simulink model "Motor_Quadcopter_Combined_Current"  (R2016b)
settings: Solver=VariableStepAuto  StartTime=0.0  StopTime=500  RelTol=1e-3
libraries: simulink x36
(part 1 of 5)
settings Model: Creator=hermansoyfer  LastModifiedBy=cskulkar

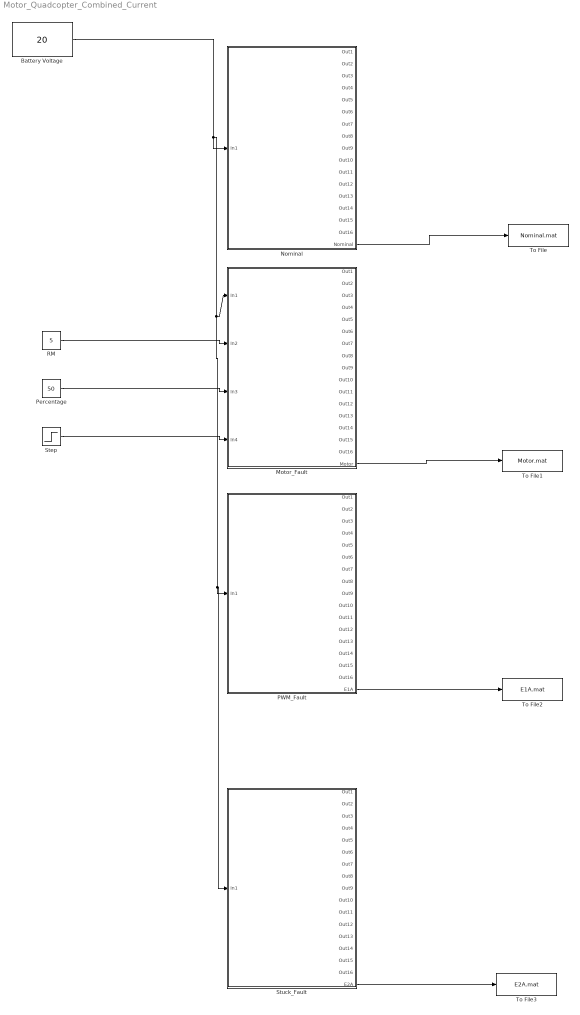
== system Motor_Quadcopter_Combined_Current ==
  Battery Voltage : Constant  Value=20
  Motor_Fault : Subsystem
  Nominal : Subsystem
  PWM_Fault : Subsystem
  Percentage : Constant  Value=50
  RM : Constant  Value=5
  Step : Step  Time=250  SampleTime=0
  Stuck_Fault : Subsystem
  To File : ToFile  Filename=Nominal.mat  MatrixName=Data
  To File1 : ToFile  Filename=Motor.mat  MatrixName=Data
  To File2 : ToFile  Filename=E1A.mat  MatrixName=Data
  To File3 : ToFile  Filename=E2A.mat  MatrixName=Data
  wires:
  Battery Voltage/1 -> Stuck_Fault/1(In1), PWM_Fault/1(In1), Motor_Fault/1(In1), Nominal/1(In1)
  Nominal/17(Nominal) -> To File/1
  Motor_Fault/17(Motor) -> To File1/1
  Percentage/1 -> Motor_Fault/3(In3)
  RM/1 -> Motor_Fault/2(In2)
  Step/1 -> Motor_Fault/4(In4)
  PWM_Fault/17(E1A) -> To File2/1
  Stuck_Fault/17(E2A) -> To File3/1

== system Motor_Quadcopter_Combined_Current/Motor_Fault ==
  In1 : Inport
  In2 : Inport  Port=2
  In3 : Inport  Port=3
  In4 : Inport  Port=4
  Add : Sum  Inputs=++++
  Add{1..4} (4 alike) : Sum
  Band-Limited White Noise1 : simulink/Sources/Band-Limited White Noise  Cov=[0.0001]  Ts=0.01  seed=[61]
  Band-Limited White Noise2 : simulink/Sources/Band-Limited White Noise  Cov=[0.0001]  Ts=0.01  seed=[678451]
  Band-Limited White Noise3 : simulink/Sources/Band-Limited White Noise  Cov=[0.0001]  Ts=0.01  seed=[95461]
  Band-Limited White Noise5 : simulink/Sources/Band-Limited White Noise  Cov=[0.0001]  Ts=0.01  seed=[34592]
  Gain : Gain  Gain=1/100
  Mux1 : Mux  Inputs=2
  Mux2 : Mux
  Mux3 : Mux
  Product : Product
  Product1 : Product
  Quadcopter_Arm1 : Subsystem
  Quadcopter_Arm3 : Subsystem
  Quadcopter_Arm4 : Subsystem
  Quatcopter_Arm2 : Subsystem
  Scope : Scope
  Scope1 : Scope  NumInputPorts=4
  Subsystem : Subsystem
  Subsystem1 : Subsystem
  Subsystem2 : Subsystem
  Subsystem3 : Subsystem
  Subsystem4 : Subsystem
  Subtract : Sum  Inputs=+-
  Out1 : Outport
  Out2 : Outport  Port=2
  Out3 : Outport  Port=3
  Out4 : Outport  Port=4
  Out5 : Outport  Port=5
  Out6 : Outport  Port=6
  Out7 : Outport  Port=7
  Out8 : Outport  Port=8
  Out9 : Outport  Port=9
  Out10 : Outport  Port=10
  Out11 : Outport  Port=11
  Out12 : Outport  Port=12
  Out13 : Outport  Port=13
  Out14 : Outport  Port=14
  Out15 : Outport  Port=15
  Out16 : Outport  Port=16
  Motor : Outport  Port=17
  wires:
  Quadcopter_Arm4/3(Out3) -> Out15/1
  Quatcopter_Arm2/4(Out4) -> Out8/1
  Quadcopter_Arm1/4(Out4) -> Out4/1
  In1/1 -> Quadcopter_Arm1/1(In1), Quatcopter_Arm2/1(In1), Quadcopter_Arm3/1(In1), Quadcopter_Arm4/1(In1)
  Quadcopter_Arm1/5(M1Current) -> Subsystem1/1(In1), Add/1
  Quatcopter_Arm2/5(M2Current) -> Subsystem2/1(In1), Add/2
  Quadcopter_Arm3/6(M3Current) -> Subsystem3/1(In1), Add/3
  Quadcopter_Arm4/6(M4Current) -> Subsystem4/1(In1), Add/4
  Quadcopter_Arm1/6(M1Voltage) -> Add1/1
  Quatcopter_Arm2/6(M2Voltatge) -> Add2/1
  Quadcopter_Arm3/5(M3Voltage) -> Add3/1
  Quadcopter_Arm4/5(M4Voltage) -> Add4/1
  Mux1/1 -> Motor/1
  Quadcopter_Arm4/4(Out4) -> Out16/1
  Quadcopter_Arm4/1(Out1) -> Out13/1
  Quadcopter_Arm4/2(Out2) -> Out14/1
  Quadcopter_Arm3/2(Out2) -> Out10/1
  Quatcopter_Arm2/2(Out2) -> Out6/1
  Quadcopter_Arm1/2(Out2) -> Out2/1
  Quadcopter_Arm3/3(Out3) -> Out11/1
  Quadcopter_Arm1/1(Out1) -> Out1/1
  Quatcopter_Arm2/3(Out3) -> Out7/1
  Quadcopter_Arm3/1(Out1) -> Out9/1
  Quatcopter_Arm2/1(Out1) -> Out5/1
  Quadcopter_Arm1/3(Out3) -> Out3/1
  Quadcopter_Arm3/4(Out4) -> Out12/1
  In4/1 -> Product1/2
  In2/1 -> Subtract/1, Product/1
  Product/1 -> Product1/1
  Product1/1 -> Subtract/2
  Subtract/1 -> Quadcopter_Arm1/2(Resistance)
  Gain/1 -> Product/2
  In3/1 -> Gain/1
  Band-Limited White Noise1/1 -> Add1/2
  Band-Limited White Noise2/1 -> Add2/2
  Band-Limited White Noise3/1 -> Add3/2
  Band-Limited White Noise5/1 -> Add4/2
  Add1/1 -> Scope1/1, Mux2/1
  Add2/1 -> Scope1/2, Mux2/2
  Add4/1 -> Scope1/4, Mux2/4
  Mux2/1 -> Mux1/1
  Subsystem/1(Out1) -> Scope/1
  Add/1 -> Subsystem/1(In1)
  Subsystem1/1(Out1) -> Mux3/1
  Subsystem2/1(Out1) -> Mux3/2
  Subsystem3/1(Out1) -> Mux3/3
  Subsystem4/1(Out1) -> Mux3/4
  Mux3/1 -> Mux1/2
  Add3/1 -> Scope1/3, Mux2/3

== system Motor_Quadcopter_Combined_Current/Nominal ==
  In1 : Inport
  Add : Sum  Inputs=++++
  Add{1..9} (9 alike) : Sum
  Band-Limited White Noise : simulink/Sources/Band-Limited White Noise  Cov=[0.0001]  Ts=0.01  seed=[23341]
  Band-Limited White Noise1 : simulink/Sources/Band-Limited White Noise  Cov=[0.0001]  Ts=0.01  seed=[322431]
  Band-Limited White Noise2 : simulink/Sources/Band-Limited White Noise  Cov=[0.0001]  Ts=0.01  seed=[685331]
  Band-Limited White Noise3 : simulink/Sources/Band-Limited White Noise  Cov=[0.0001]  Ts=0.01  seed=[456]
  Band-Limited White Noise4 : simulink/Sources/Band-Limited White Noise  Cov=[0.0001]  Ts=0.01  seed=[25561]
  Band-Limited White Noise5 : simulink/Sources/Band-Limited White Noise  Cov=[0.0001]  Ts=0.01  seed=[55321]
  Band-Limited White Noise6 : simulink/Sources/Band-Limited White Noise  Cov=[0.0005]  Ts=0.01  seed=[3452]
  Band-Limited White Noise7 : simulink/Sources/Band-Limited White Noise  Cov=[0.0002]  Ts=0.01  seed=[255]
  Band-Limited White Noise8 : simulink/Sources/Band-Limited White Noise  Cov=[0.0001]  Ts=0.01  seed=[61244]
  Mux : Mux
  Mux1 : Mux  Inputs=2
  Mux2 : Mux
  Quadcopter_Arm1 : Subsystem
  Quadcopter_Arm3 : Subsystem
  Quadcopter_Arm4 : Subsystem
  Quatcopter_Arm2 : Subsystem
  Scope : Scope
  Scope1 : Scope
  Scope2 : Scope
  Out1 : Outport
  Out2 : Outport  Port=2
  Out3 : Outport  Port=3
  Out4 : Outport  Port=4
  Out5 : Outport  Port=5
  Out6 : Outport  Port=6
  Out7 : Outport  Port=7
  Out8 : Outport  Port=8
  Out9 : Outport  Port=9
  Out10 : Outport  Port=10
  Out11 : Outport  Port=11
  Out12 : Outport  Port=12
  Out13 : Outport  Port=13
  Out14 : Outport  Port=14
  Out15 : Outport  Port=15
  Out16 : Outport  Port=16
  Nominal : Outport  Port=17
  wires:
  Quadcopter_Arm4/3(Out3) -> Out15/1
  Quatcopter_Arm2/4(Out4) -> Out8/1
  Quadcopter_Arm1/4(Out4) -> Out4/1
  In1/1 -> Quadcopter_Arm1/1(In1), Quatcopter_Arm2/1(In1), Quadcopter_Arm3/1(In1), Quadcopter_Arm4/1(In1)
  Quadcopter_Arm1/5(M1Current) -> Add6/1, Add/1
  Quatcopter_Arm2/5(M2Current) -> Add7/1, Add/2
  Quadcopter_Arm3/6(M3Current) -> Add9/1, Add8/1, Add/3
  Quadcopter_Arm4/6(M4Current) -> Add/4
  Quadcopter_Arm1/6(M1Voltage) -> Add1/1
  Quatcopter_Arm2/6(M2Voltatge) -> Add2/1
  Quadcopter_Arm3/5(M3Voltage) -> Add3/2
  Quadcopter_Arm4/5(M4Voltage) -> Add4/1
  Mux1/1 -> Nominal/1
  Quadcopter_Arm4/4(Out4) -> Out16/1
  Quadcopter_Arm4/1(Out1) -> Out13/1
  Quadcopter_Arm4/2(Out2) -> Out14/1
  Quadcopter_Arm3/2(Out2) -> Out10/1
  Quatcopter_Arm2/2(Out2) -> Out6/1
  Quadcopter_Arm1/2(Out2) -> Out2/1
  Quadcopter_Arm3/3(Out3) -> Out11/1
  Quadcopter_Arm1/1(Out1) -> Out1/1
  Quatcopter_Arm2/3(Out3) -> Out7/1
  Quadcopter_Arm3/1(Out1) -> Out9/1
  Quatcopter_Arm2/1(Out1) -> Out5/1
  Quadcopter_Arm1/3(Out3) -> Out3/1
  Quadcopter_Arm3/4(Out4) -> Out12/1
  Band-Limited White Noise/1 -> Add1/2
  Band-Limited White Noise1/1 -> Add2/2
  Band-Limited White Noise2/1 -> Add3/1
  Add1/1 -> Mux/1
  Add2/1 -> Mux/2
  Add3/1 -> Mux/3
  Add4/1 -> Mux/4
  Mux/1 -> Scope/1, Mux1/1
  Add/1 -> Add5/1
  Band-Limited White Noise4/1 -> Add5/2
  Add5/1 -> Scope1/1
  Band-Limited White Noise3/1 -> Add4/2
  Band-Limited White Noise5/1 -> Add6/2
  Add6/1 -> Mux2/1
  Band-Limited White Noise6/1 -> Add7/2
  Add7/1 -> Mux2/2
  Band-Limited White Noise7/1 -> Add8/2
  Add8/1 -> Mux2/3
  Add9/1 -> Mux2/4
  Band-Limited White Noise8/1 -> Add9/2
  Mux2/1 -> Scope2/1, Mux1/2

== system Motor_Quadcopter_Combined_Current/PWM_Fault ==
  In1 : Inport
  Add : Sum  Inputs=++++
  Add{1..4} (4 alike) : Sum
  Band-Limited White Noise{1..3,5} (4 alike) : simulink/Sources/Band-Limited White Noise  Cov=[0.0001]  Ts=0.01  seed=[46561]
  Mux1 : Mux  Inputs=2
  Mux2 : Mux
  Mux3 : Mux
  Quadcopter_Arm1 : Subsystem
  Quadcopter_Arm3 : Subsystem
  Quadcopter_Arm4 : Subsystem
  Quatcopter_Arm2 : Subsystem
  Scope : Scope
  Scope1 : Scope
  Subsystem : Subsystem
  Subsystem1 : Subsystem
  Subsystem2 : Subsystem
  Subsystem3 : Subsystem
  Subsystem4 : Subsystem
  Out1 : Outport
  Out2 : Outport  Port=2
  Out3 : Outport  Port=3
  Out4 : Outport  Port=4
  Out5 : Outport  Port=5
  Out6 : Outport  Port=6
  Out7 : Outport  Port=7
  Out8 : Outport  Port=8
  Out9 : Outport  Port=9
  Out10 : Outport  Port=10
  Out11 : Outport  Port=11
  Out12 : Outport  Port=12
  Out13 : Outport  Port=13
  Out14 : Outport  Port=14
  Out15 : Outport  Port=15
  Out16 : Outport  Port=16
  E1A : Outport  Port=17
  wires:
  Quadcopter_Arm4/3(Out3) -> Out15/1
  Quatcopter_Arm2/4(Out4) -> Out8/1
  Quadcopter_Arm1/4(Out4) -> Out4/1
  In1/1 -> Quadcopter_Arm1/1(In1), Quatcopter_Arm2/1(In1), Quadcopter_Arm3/1(In1), Quadcopter_Arm4/1(In1)
  Quadcopter_Arm1/5(M1Current) -> Subsystem1/1(In1), Add/1
  Quatcopter_Arm2/5(M2Current) -> Subsystem2/1(In1), Add/2
  Quadcopter_Arm3/6(M3Current) -> Subsystem3/1(In1), Add/3
  Quadcopter_Arm4/6(M4Current) -> Subsystem4/1(In1), Add/4
  Quadcopter_Arm1/6(M1Voltage) -> Add1/1
  Quatcopter_Arm2/6(M2Voltatge) -> Add2/1
  Quadcopter_Arm3/5(M3Voltage) -> Add3/1
  Quadcopter_Arm4/5(M4Voltage) -> Add4/1
  Mux1/1 -> E1A/1
  Quadcopter_Arm4/4(Out4) -> Out16/1
  Quadcopter_Arm4/1(Out1) -> Out13/1
  Quadcopter_Arm4/2(Out2) -> Out14/1
  Quadcopter_Arm3/2(Out2) -> Out10/1
  Quatcopter_Arm2/2(Out2) -> Out6/1
  Quadcopter_Arm1/2(Out2) -> Out2/1
  Quadcopter_Arm3/3(Out3) -> Out11/1
  Quadcopter_Arm1/1(Out1) -> Out1/1
  Quatcopter_Arm2/3(Out3) -> Out7/1
  Quadcopter_Arm3/1(Out1) -> Out9/1
  Quatcopter_Arm2/1(Out1) -> Out5/1
  Quadcopter_Arm1/3(Out3) -> Out3/1
  Quadcopter_Arm3/4(Out4) -> Out12/1
  Band-Limited White Noise1/1 -> Add1/2
  Band-Limited White Noise2/1 -> Add2/2
  Band-Limited White Noise3/1 -> Add3/2
  Band-Limited White Noise5/1 -> Add4/2
  Add1/1 -> Mux2/1
  Add2/1 -> Mux2/2
  Add3/1 -> Mux2/3
  Mux2/1 -> Scope/1, Mux1/1
  Add4/1 -> Mux2/4
  Subsystem/1(Out1) -> Scope1/1
  Add/1 -> Subsystem/1(In1)
  Subsystem1/1(Out1) -> Mux3/1
  Subsystem2/1(Out1) -> Mux3/2
  Subsystem3/1(Out1) -> Mux3/3
  Subsystem4/1(Out1) -> Mux3/4
  Mux3/1 -> Mux1/2

== system Motor_Quadcopter_Combined_Current/Stuck_Fault ==
  In1 : Inport
  Add : Sum  Inputs=++++
  Add{1..4} (4 alike) : Sum
  Band-Limited White Noise1 : simulink/Sources/Band-Limited White Noise  Cov=[0.0001]  Ts=0.01  seed=[678]
  Band-Limited White Noise2 : simulink/Sources/Band-Limited White Noise  Cov=[0.0001]  Ts=0.01  seed=[1111]
  Band-Limited White Noise3 : simulink/Sources/Band-Limited White Noise  Cov=[0.0001]  Ts=0.01  seed=[61]
  Band-Limited White Noise5 : simulink/Sources/Band-Limited White Noise  Cov=[0.0001]  Ts=0.01  seed=[4]
  Mux1 : Mux  Inputs=2
  Mux2 : Mux
  Mux3 : Mux
  Quadcopter_Arm1 : Subsystem
  Quadcopter_Arm3 : Subsystem
  Quadcopter_Arm4 : Subsystem
  Quatcopter_Arm2 : Subsystem
  Scope : Scope
  Scope1 : Scope
  Scope2 : Scope  NumInputPorts=4
  Subsystem : Subsystem
  Subsystem1 : Subsystem
  Subsystem2 : Subsystem
  Subsystem3 : Subsystem
  Subsystem4 : Subsystem
  Out1 : Outport
  Out2 : Outport  Port=2
  Out3 : Outport  Port=3
  Out4 : Outport  Port=4
  Out5 : Outport  Port=5
  Out6 : Outport  Port=6
  Out7 : Outport  Port=7
  Out8 : Outport  Port=8
  Out9 : Outport  Port=9
  Out10 : Outport  Port=10
  Out11 : Outport  Port=11
  Out12 : Outport  Port=12
  Out13 : Outport  Port=13
  Out14 : Outport  Port=14
  Out15 : Outport  Port=15
  Out16 : Outport  Port=16
  E2A : Outport  Port=17
  wires:
  Quadcopter_Arm4/3(Out3) -> Out15/1
  Quatcopter_Arm2/4(Out4) -> Out8/1
  Quadcopter_Arm1/4(Out4) -> Out4/1
  In1/1 -> Quadcopter_Arm1/1(In1), Quatcopter_Arm2/1(In1), Quadcopter_Arm3/1(In1), Quadcopter_Arm4/1(In1)
  Quadcopter_Arm1/5(M1Current) -> Subsystem1/1(In1), Add/1
  Quatcopter_Arm2/5(M2Current) -> Subsystem2/1(In1), Add/2
  Quadcopter_Arm3/6(M3Current) -> Subsystem3/1(In1), Add/3
  Quadcopter_Arm4/6(M4Current) -> Subsystem4/1(In1), Add/4
  Quadcopter_Arm1/6(M1Voltage) -> Add1/1
  Quadcopter_Arm4/4(Out4) -> Out16/1
  Quadcopter_Arm4/1(Out1) -> Out13/1
  Quadcopter_Arm4/2(Out2) -> Out14/1
  Quadcopter_Arm3/2(Out2) -> Out10/1
  Quatcopter_Arm2/2(Out2) -> Out6/1
  Quadcopter_Arm1/2(Out2) -> Out2/1
  Quadcopter_Arm3/3(Out3) -> Out11/1
  Quadcopter_Arm1/1(Out1) -> Out1/1
  Quatcopter_Arm2/3(Out3) -> Out7/1
  Quadcopter_Arm3/1(Out1) -> Out9/1
  Quatcopter_Arm2/1(Out1) -> Out5/1
  Quadcopter_Arm1/3(Out3) -> Out3/1
  Quadcopter_Arm3/4(Out4) -> Out12/1
  Band-Limited White Noise1/1 -> Add1/2
  Band-Limited White Noise2/1 -> Add2/2
  Band-Limited White Noise3/1 -> Add3/2
  Band-Limited White Noise5/1 -> Add4/2
  Quatcopter_Arm2/6(M2Voltatge) -> Add2/1
  Quadcopter_Arm3/5(M3Voltage) -> Add3/1
  Quadcopter_Arm4/5(M4Voltage) -> Add4/1
  Add1/1 -> Mux2/1
  Add2/1 -> Mux2/2
  Add3/1 -> Mux2/3
  Add4/1 -> Mux2/4
  Mux2/1 -> Mux1/1
  Mux1/1 -> Scope/1, E2A/1
  Subsystem/1(Out1) -> Scope1/1
  Add/1 -> Subsystem/1(In1)
  Subsystem1/1(Out1) -> Scope2/2, Mux3/1
  Subsystem2/1(Out1) -> Scope2/1, Mux3/2
  Subsystem3/1(Out1) -> Scope2/3, Mux3/3
  Subsystem4/1(Out1) -> Scope2/4, Mux3/4
  Mux3/1 -> Mux1/2

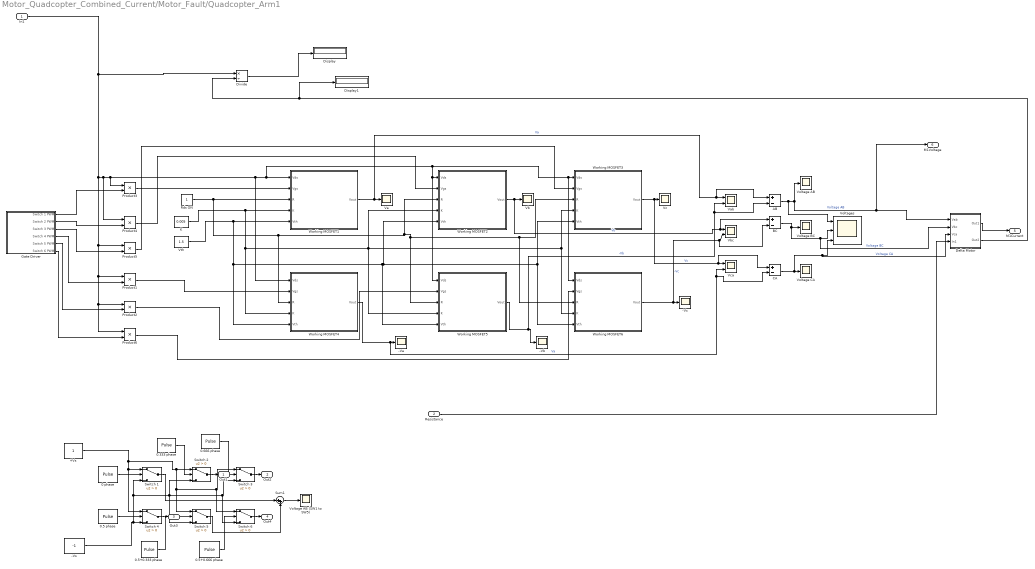
== system Motor_Quadcopter_Combined_Current/Motor_Fault/Quadcopter_Arm1 ==
  In1 : Inport
  Resistance : Inport  Port=2
  +Vs : Constant
  -Va : Scope
  -Vb : Scope
  -Vc : Scope
  -Vs : Constant  Value=-1
  0 phase : DiscretePulseGenerator  PulseType=Time based  Period=1  PulseWidth=50
  0.333 phase : DiscretePulseGenerator  PulseType=Time based  Period=1  PulseWidth=50  PhaseDelay=1/3
  0.5 phase : DiscretePulseGenerator  PulseType=Time based  Period=1  PulseWidth=50  PhaseDelay=.5
  0.5+0.333 phase : DiscretePulseGenerator  PulseType=Time based  Period=1  PulseWidth=50  PhaseDelay=0.5 + 1/3
  0.5+0.666 phase : DiscretePulseGenerator  PulseType=Time based  Period=1  PulseWidth=50  PhaseDelay=2/3+0.5
  0.666 phase : DiscretePulseGenerator  PulseType=Time based  Period=1  PulseWidth=50  PhaseDelay=2/3
  AB : Sum  Inputs=+-
  BC : Sum  Inputs=+-
  CA : Sum  Inputs=+-
  Delta Motor : Subsystem
  Display : Display
  Display1 : Display
  Divide : Product  Inputs=*/
  Gate Driver : Subsystem
  K : Constant  Value=0.005
  Product{1..6} (6 alike) : Product
  Rds ON : Constant
  Sum1 : Sum  Inputs=|++
  Switch {1..6} (6 alike) : Switch  Criteria=u2 > Threshold
  Va : Scope
  Vab : Scope  NumInputPorts=2
  Vb : Scope
  Vbc : Scope  NumInputPorts=2
  Vc : Scope
  Vca : Scope  NumInputPorts=2
  Voltage AB : Scope
  Voltage AB (SW1 to SW5) : Scope
  Voltage BC : Scope
  Voltage CA : Scope
  Voltages : Scope  NumInputPorts=3
  Vth : Constant  Value=1.5
  Working MOSFET1 : MATLAB Function  TreatAsAtomicUnit=on
  Working MOSFET2 : MATLAB Function  TreatAsAtomicUnit=on
  Working MOSFET3 : MATLAB Function  TreatAsAtomicUnit=on
  Working MOSFET4 : MATLAB Function  TreatAsAtomicUnit=on
  Working MOSFET5 : MATLAB Function  TreatAsAtomicUnit=on
  Working MOSFET6 : MATLAB Function  TreatAsAtomicUnit=on
  Out1 : Outport
  Out2 : Outport  Port=2
  Out3 : Outport  Port=3
  Out4 : Outport  Port=4
  M1Current : Outport  Port=5
  M1Voltage : Outport  Port=6
  wires:
  Switch 5/1 -> Sum1/2
  Working MOSFET4/1(Vout) -> CA/2, Vca/2, -Va/1  "Va"
  Working MOSFET6/1(Vout) -> BC/2, Vbc/2, -Vc/1  "-Vc"
  AB/1 -> Voltages/1, M1Voltage/1, Delta Motor/1(Vab), Voltage AB/1  "Voltage AB"
  In1/1 -> Divide/1, Product6/1, Product2/1, Product1/1, Product5/1, Product4/1, Working MOSFET4/1(Vds), Working MOSFET6/1(Vds), Working MOSFET3/1(Vds), Working MOSFET5/1(Vds), Working MOSFET2/1(Vds), Working MOSFET1/1(Vds), Product3/1
  K/1 -> Working MOSFET4/4(K), Working MOSFET5/4(K), Working MOSFET2/4(K), Working MOSFET6/4(K), Working MOSFET3/4(K), Working MOSFET1/4(K)
  Product5/1 -> Working MOSFET3/2(Vgs)
  0.5+0.333 phase/1 -> Switch 5/2
  Gate Driver/3(Switch 3 PWM) -> Product5/2
  Gate Driver/6(Switch 6 PWM) -> Product6/2
  Working MOSFET5/1(Vout) -> AB/2, Vab/2, -Vb/1  "-Vb"
  Gate Driver/5(Switch 5 PWM) -> Product2/2
  Working MOSFET1/1(Vout) -> AB/1, Vab/1, Va/1  "Va"
  0 phase/1 -> Switch 1/2
  Gate Driver/2(Switch 2 PWM) -> Product4/2
  Gate Driver/4(Switch 4 PWM) -> Product1/2
  BC/1 -> Delta Motor/2(Vbc), Voltages/2, Voltage BC/1  "Voltage BC"
  CA/1 -> Delta Motor/3(Vca), Voltages/3, Voltage CA/1  "Voltage CA"
  Working MOSFET3/1(Vout) -> CA/1, Vca/1, Vc/1  "Vc"
  Gate Driver/1(Switch 1 PWM) -> Product3/2
  Vth/1 -> Working MOSFET4/5(Vth), Working MOSFET5/5(Vth), Working MOSFET2/5(Vth), Working MOSFET6/5(Vth), Working MOSFET3/5(Vth), Working MOSFET1/5(Vth)
  Product1/1 -> Working MOSFET4/2(Vgs)
  0.333 phase/1 -> Switch 2/2
  Sum1/1 -> Voltage AB (SW1 to SW5)/1
  0.5 phase/1 -> Switch 4/2
  Switch 1/1 -> Sum1/1
  Working MOSFET2/1(Vout) -> BC/1, Vbc/1, Vb/1  "Vb"
  Switch 6/1 -> Out4/1
  Switch 2/1 -> Out1/1
  Switch 4/1 -> Out3/1
  Product2/1 -> Working MOSFET5/2(Vgs)
  Switch 3/1 -> Out2/1
  +Vs/1 -> Switch 6/1, Switch 3/1, Switch 5/1, Switch 2/1, Switch 4/1, Switch 1/1
  0.666 phase/1 -> Switch 3/2
  0.5+0.666 phase/1 -> Switch 6/2
  -Vs/1 -> Switch 1/3, Switch 6/3, Switch 3/3, Switch 2/3, Switch 5/3, Switch 4/3
  Rds ON/1 -> Working MOSFET1/3(R), Working MOSFET4/3(R), Working MOSFET3/3(R), Working MOSFET6/3(R), Working MOSFET5/3(R), Working MOSFET2/3(R)
  Product4/1 -> Working MOSFET2/2(Vgs)
  Product3/1 -> Working MOSFET1/2(Vgs)
  Product6/1 -> Working MOSFET6/2(Vgs)
  Delta Motor/1(Out1) -> M1Current/1
  Divide/1 -> Display/1
  Delta Motor/2(Out2) -> Display1/1, Divide/2
  Resistance/1 -> Delta Motor/4(In1)

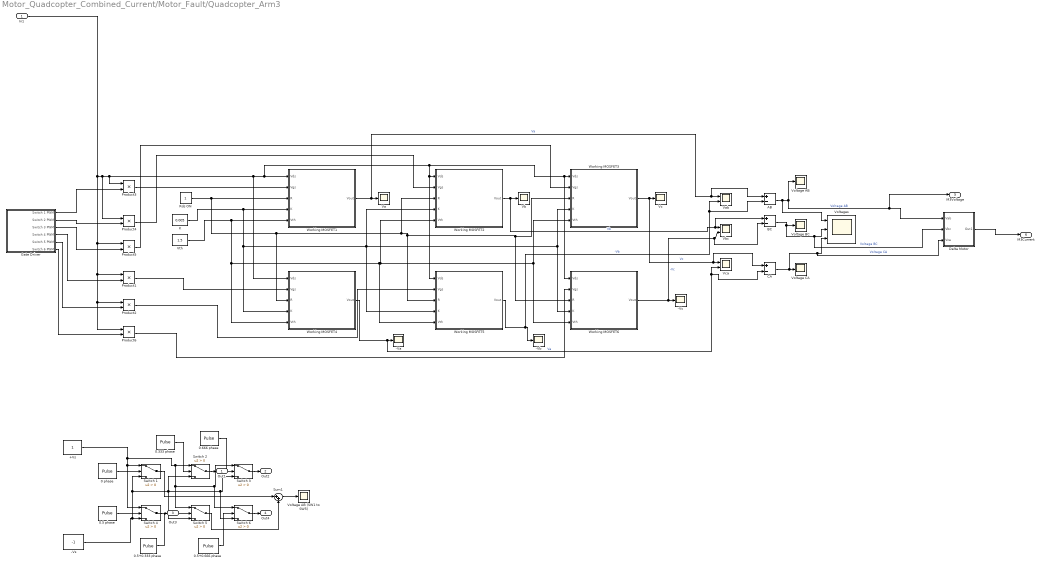
== system Motor_Quadcopter_Combined_Current/Motor_Fault/Quadcopter_Arm3 ==
  In1 : Inport
  +Vs : Constant
  -Va : Scope
  -Vb : Scope
  -Vc : Scope
  -Vs : Constant  Value=-1
  0 phase : DiscretePulseGenerator  PulseType=Time based  Period=1  PulseWidth=50
  0.333 phase : DiscretePulseGenerator  PulseType=Time based  Period=1  PulseWidth=50  PhaseDelay=1/3
  0.5 phase : DiscretePulseGenerator  PulseType=Time based  Period=1  PulseWidth=50  PhaseDelay=.5
  0.5+0.333 phase : DiscretePulseGenerator  PulseType=Time based  Period=1  PulseWidth=50  PhaseDelay=0.5 + 1/3
  0.5+0.666 phase : DiscretePulseGenerator  PulseType=Time based  Period=1  PulseWidth=50  PhaseDelay=2/3+0.5
  0.666 phase : DiscretePulseGenerator  PulseType=Time based  Period=1  PulseWidth=50  PhaseDelay=2/3
  AB : Sum  Inputs=+-
  BC : Sum  Inputs=+-
  CA : Sum  Inputs=+-
  Delta Motor : Subsystem
  Gate Driver : Subsystem
  K : Constant  Value=0.005
  Product{1..6} (6 alike) : Product
  Rds ON : Constant
  Sum1 : Sum  Inputs=|++
  Switch {1..6} (6 alike) : Switch  Criteria=u2 > Threshold
  Va : Scope
  Vab : Scope  NumInputPorts=2
  Vb : Scope
  Vbc : Scope  NumInputPorts=2
  Vc : Scope
  Vca : Scope  NumInputPorts=2
  Voltage AB : Scope
  Voltage AB (SW1 to SW5) : Scope
  Voltage BC : Scope
  Voltage CA : Scope
  Voltages : Scope  NumInputPorts=3
  Vth : Constant  Value=1.5
  Working MOSFET1 : MATLAB Function  TreatAsAtomicUnit=on
  Working MOSFET2 : MATLAB Function  TreatAsAtomicUnit=on
  Working MOSFET3 : MATLAB Function  TreatAsAtomicUnit=on
  Working MOSFET4 : MATLAB Function  TreatAsAtomicUnit=on
  Working MOSFET5 : MATLAB Function  TreatAsAtomicUnit=on
  Working MOSFET6 : MATLAB Function  TreatAsAtomicUnit=on
  Out1 : Outport
  Out2 : Outport  Port=2
  Out3 : Outport  Port=3
  Out4 : Outport  Port=4
  M3Voltage : Outport  Port=5
  M3Current : Outport  Port=6
  wires:
  Switch 5/1 -> Sum1/2
  Working MOSFET4/1(Vout) -> CA/2, Vca/2, -Va/1  "Va"
  Working MOSFET6/1(Vout) -> BC/2, Vbc/2, -Vc/1  "-Vc"
  AB/1 -> Voltages/1, M3Voltage/1, Delta Motor/1(Vab), Voltage AB/1  "Voltage AB"
  In1/1 -> Product6/1, Product2/1, Product1/1, Product5/1, Product4/1, Working MOSFET4/1(Vds), Working MOSFET6/1(Vds), Working MOSFET3/1(Vds), Working MOSFET5/1(Vds), Working MOSFET2/1(Vds), Working MOSFET1/1(Vds), Product3/1
  K/1 -> Working MOSFET4/4(K), Working MOSFET5/4(K), Working MOSFET2/4(K), Working MOSFET6/4(K), Working MOSFET3/4(K), Working MOSFET1/4(K)
  Product5/1 -> Working MOSFET3/2(Vgs)
  0.5+0.333 phase/1 -> Switch 5/2
  Gate Driver/3(Switch 3 PWM) -> Product5/2
  Gate Driver/6(Switch 6 PWM) -> Product6/2
  Working MOSFET5/1(Vout) -> AB/2, Vab/2, -Vb/1  "-Vb"
  Gate Driver/5(Switch 5 PWM) -> Product2/2
  Working MOSFET1/1(Vout) -> AB/1, Vab/1, Va/1  "Va"
  0 phase/1 -> Switch 1/2
  Gate Driver/2(Switch 2 PWM) -> Product4/2
  Gate Driver/4(Switch 4 PWM) -> Product1/2
  BC/1 -> Delta Motor/2(Vbc), Voltages/2, Voltage BC/1  "Voltage BC"
  CA/1 -> Delta Motor/3(Vca), Voltages/3, Voltage CA/1  "Voltage CA"
  Working MOSFET3/1(Vout) -> CA/1, Vca/1, Vc/1  "Vc"
  Gate Driver/1(Switch 1 PWM) -> Product3/2
  Vth/1 -> Working MOSFET4/5(Vth), Working MOSFET5/5(Vth), Working MOSFET2/5(Vth), Working MOSFET6/5(Vth), Working MOSFET3/5(Vth), Working MOSFET1/5(Vth)
  Product1/1 -> Working MOSFET4/2(Vgs)
  0.333 phase/1 -> Switch 2/2
  Sum1/1 -> Voltage AB (SW1 to SW5)/1
  0.5 phase/1 -> Switch 4/2
  Switch 1/1 -> Sum1/1
  Working MOSFET2/1(Vout) -> BC/1, Vbc/1, Vb/1  "Vb"
  Switch 6/1 -> Out4/1
  Switch 2/1 -> Out1/1
  Switch 4/1 -> Out3/1
  Product2/1 -> Working MOSFET5/2(Vgs)
  Switch 3/1 -> Out2/1
  +Vs/1 -> Switch 6/1, Switch 3/1, Switch 5/1, Switch 2/1, Switch 4/1, Switch 1/1
  0.666 phase/1 -> Switch 3/2
  0.5+0.666 phase/1 -> Switch 6/2
  -Vs/1 -> Switch 1/3, Switch 6/3, Switch 3/3, Switch 2/3, Switch 5/3, Switch 4/3
  Rds ON/1 -> Working MOSFET1/3(R), Working MOSFET4/3(R), Working MOSFET3/3(R), Working MOSFET6/3(R), Working MOSFET5/3(R), Working MOSFET2/3(R)
  Product4/1 -> Working MOSFET2/2(Vgs)
  Product3/1 -> Working MOSFET1/2(Vgs)
  Product6/1 -> Working MOSFET6/2(Vgs)
  Delta Motor/1(Out1) -> M3Current/1

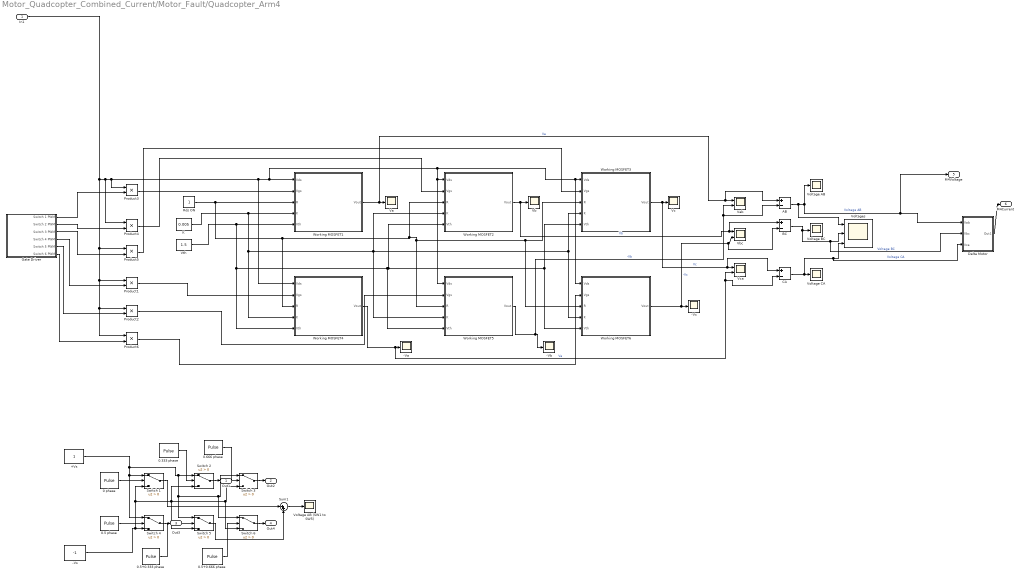
== system Motor_Quadcopter_Combined_Current/Motor_Fault/Quadcopter_Arm4 ==
  In1 : Inport
  +Vs : Constant
  -Va : Scope
  -Vb : Scope
  -Vc : Scope
  -Vs : Constant  Value=-1
  0 phase : DiscretePulseGenerator  PulseType=Time based  Period=1  PulseWidth=50
  0.333 phase : DiscretePulseGenerator  PulseType=Time based  Period=1  PulseWidth=50  PhaseDelay=1/3
  0.5 phase : DiscretePulseGenerator  PulseType=Time based  Period=1  PulseWidth=50  PhaseDelay=.5
  0.5+0.333 phase : DiscretePulseGenerator  PulseType=Time based  Period=1  PulseWidth=50  PhaseDelay=0.5 + 1/3
  0.5+0.666 phase : DiscretePulseGenerator  PulseType=Time based  Period=1  PulseWidth=50  PhaseDelay=2/3+0.5
  0.666 phase : DiscretePulseGenerator  PulseType=Time based  Period=1  PulseWidth=50  PhaseDelay=2/3
  AB : Sum  Inputs=+-
  BC : Sum  Inputs=+-
  CA : Sum  Inputs=+-
  Delta Motor : Subsystem
  Gate Driver : Subsystem
  K : Constant  Value=0.005
  Product{1..6} (6 alike) : Product
  Rds ON : Constant
  Sum1 : Sum  Inputs=|++
  Switch {1..6} (6 alike) : Switch  Criteria=u2 > Threshold
  Va : Scope
  Vab : Scope  NumInputPorts=2
  Vb : Scope
  Vbc : Scope  NumInputPorts=2
  Vc : Scope
  Vca : Scope  NumInputPorts=2
  Voltage AB : Scope
  Voltage AB (SW1 to SW5) : Scope
  Voltage BC : Scope
  Voltage CA : Scope
  Voltages : Scope  NumInputPorts=3
  Vth : Constant  Value=1.5
  Working MOSFET1 : MATLAB Function  TreatAsAtomicUnit=on
  Working MOSFET2 : MATLAB Function  TreatAsAtomicUnit=on
  Working MOSFET3 : MATLAB Function  TreatAsAtomicUnit=on
  Working MOSFET4 : MATLAB Function  TreatAsAtomicUnit=on
  Working MOSFET5 : MATLAB Function  TreatAsAtomicUnit=on
  Working MOSFET6 : MATLAB Function  TreatAsAtomicUnit=on
  Out1 : Outport
  Out2 : Outport  Port=2
  Out3 : Outport  Port=3
  Out4 : Outport  Port=4
  M4Voltage : Outport  Port=5
  M4Current : Outport  Port=6
  wires:
  Switch 5/1 -> Sum1/2
  Working MOSFET4/1(Vout) -> CA/2, Vca/2, -Va/1  "Va"
  Working MOSFET6/1(Vout) -> BC/2, Vbc/2, -Vc/1  "-Vc"
  AB/1 -> Voltages/1, M4Voltage/1, Delta Motor/1(Vab), Voltage AB/1  "Voltage AB"
  In1/1 -> Product6/1, Product2/1, Product1/1, Product5/1, Product4/1, Working MOSFET4/1(Vds), Working MOSFET6/1(Vds), Working MOSFET3/1(Vds), Working MOSFET5/1(Vds), Working MOSFET2/1(Vds), Working MOSFET1/1(Vds), Product3/1
  K/1 -> Working MOSFET4/4(K), Working MOSFET5/4(K), Working MOSFET2/4(K), Working MOSFET6/4(K), Working MOSFET3/4(K), Working MOSFET1/4(K)
  Product5/1 -> Working MOSFET3/2(Vgs)
  0.5+0.333 phase/1 -> Switch 5/2
  Gate Driver/3(Switch 3 PWM) -> Product5/2
  Gate Driver/6(Switch 6 PWM) -> Product6/2
  Working MOSFET5/1(Vout) -> AB/2, Vab/2, -Vb/1  "-Vb"
  Gate Driver/5(Switch 5 PWM) -> Product2/2
  Working MOSFET1/1(Vout) -> AB/1, Vab/1, Va/1  "Va"
  0 phase/1 -> Switch 1/2
  Gate Driver/2(Switch 2 PWM) -> Product4/2
  Gate Driver/4(Switch 4 PWM) -> Product1/2
  BC/1 -> Delta Motor/2(Vbc), Voltages/2, Voltage BC/1  "Voltage BC"
  CA/1 -> Delta Motor/3(Vca), Voltages/3, Voltage CA/1  "Voltage CA"
  Working MOSFET3/1(Vout) -> CA/1, Vca/1, Vc/1  "Vc"
  Gate Driver/1(Switch 1 PWM) -> Product3/2
  Vth/1 -> Working MOSFET4/5(Vth), Working MOSFET5/5(Vth), Working MOSFET2/5(Vth), Working MOSFET6/5(Vth), Working MOSFET3/5(Vth), Working MOSFET1/5(Vth)
  Product1/1 -> Working MOSFET4/2(Vgs)
  0.333 phase/1 -> Switch 2/2
  Sum1/1 -> Voltage AB (SW1 to SW5)/1
  0.5 phase/1 -> Switch 4/2
  Switch 1/1 -> Sum1/1
  Working MOSFET2/1(Vout) -> BC/1, Vbc/1, Vb/1  "Vb"
  Switch 6/1 -> Out4/1
  Switch 2/1 -> Out1/1
  Switch 4/1 -> Out3/1
  Product2/1 -> Working MOSFET5/2(Vgs)
  Switch 3/1 -> Out2/1
  +Vs/1 -> Switch 6/1, Switch 3/1, Switch 5/1, Switch 2/1, Switch 4/1, Switch 1/1
  0.666 phase/1 -> Switch 3/2
  0.5+0.666 phase/1 -> Switch 6/2
  -Vs/1 -> Switch 1/3, Switch 6/3, Switch 3/3, Switch 2/3, Switch 5/3, Switch 4/3
  Rds ON/1 -> Working MOSFET1/3(R), Working MOSFET4/3(R), Working MOSFET3/3(R), Working MOSFET6/3(R), Working MOSFET5/3(R), Working MOSFET2/3(R)
  Product4/1 -> Working MOSFET2/2(Vgs)
  Product3/1 -> Working MOSFET1/2(Vgs)
  Product6/1 -> Working MOSFET6/2(Vgs)
  Delta Motor/1(Out1) -> M4Current/1

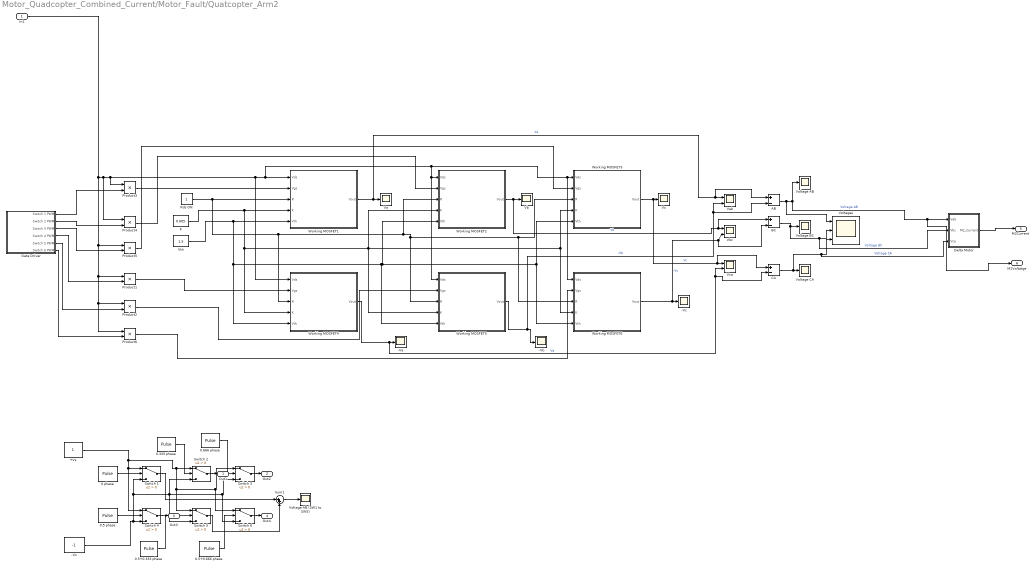
== system Motor_Quadcopter_Combined_Current/Motor_Fault/Quatcopter_Arm2 ==
  In1 : Inport
  +Vs : Constant
  -Va : Scope
  -Vb : Scope
  -Vc : Scope
  -Vs : Constant  Value=-1
  0 phase : DiscretePulseGenerator  PulseType=Time based  Period=1  PulseWidth=50
  0.333 phase : DiscretePulseGenerator  PulseType=Time based  Period=1  PulseWidth=50  PhaseDelay=1/3
  0.5 phase : DiscretePulseGenerator  PulseType=Time based  Period=1  PulseWidth=50  PhaseDelay=.5
  0.5+0.333 phase : DiscretePulseGenerator  PulseType=Time based  Period=1  PulseWidth=50  PhaseDelay=0.5 + 1/3
  0.5+0.666 phase : DiscretePulseGenerator  PulseType=Time based  Period=1  PulseWidth=50  PhaseDelay=2/3+0.5
  0.666 phase : DiscretePulseGenerator  PulseType=Time based  Period=1  PulseWidth=50  PhaseDelay=2/3
  AB : Sum  Inputs=+-
  BC : Sum  Inputs=+-
  CA : Sum  Inputs=+-
  Delta Motor : Subsystem
  Gate Driver : Subsystem
  K : Constant  Value=0.005
  Product{1..6} (6 alike) : Product
  Rds ON : Constant
  Sum1 : Sum  Inputs=|++
  Switch {1..6} (6 alike) : Switch  Criteria=u2 > Threshold
  Va : Scope
  Vab : Scope  NumInputPorts=2
  Vb : Scope
  Vbc : Scope  NumInputPorts=2
  Vc : Scope
  Vca : Scope  NumInputPorts=2
  Voltage AB : Scope
  Voltage AB (SW1 to SW5) : Scope
  Voltage BC : Scope
  Voltage CA : Scope
  Voltages : Scope  NumInputPorts=3
  Vth : Constant  Value=1.5
  Working MOSFET1 : MATLAB Function  TreatAsAtomicUnit=on
  Working MOSFET2 : MATLAB Function  TreatAsAtomicUnit=on
  Working MOSFET3 : MATLAB Function  TreatAsAtomicUnit=on
  Working MOSFET4 : MATLAB Function  TreatAsAtomicUnit=on
  Working MOSFET5 : MATLAB Function  TreatAsAtomicUnit=on
  Working MOSFET6 : MATLAB Function  TreatAsAtomicUnit=on
  Out1 : Outport
  Out2 : Outport  Port=2
  Out3 : Outport  Port=3
  Out4 : Outport  Port=4
  M2Current : Outport  Port=5
  M2Voltatge : Outport  Port=6
  wires:
  Switch 5/1 -> Sum1/2
  Working MOSFET4/1(Vout) -> CA/2, Vca/2, -Va/1  "Va"
  Working MOSFET6/1(Vout) -> BC/2, Vbc/2, -Vc/1  "-Vc"
  AB/1 -> Voltages/1, M2Voltatge/1, Delta Motor/1(Vab), Voltage AB/1  "Voltage AB"
  In1/1 -> Product6/1, Product2/1, Product1/1, Product5/1, Product4/1, Working MOSFET4/1(Vds), Working MOSFET6/1(Vds), Working MOSFET3/1(Vds), Working MOSFET5/1(Vds), Working MOSFET2/1(Vds), Working MOSFET1/1(Vds), Product3/1
  K/1 -> Working MOSFET4/4(K), Working MOSFET5/4(K), Working MOSFET2/4(K), Working MOSFET6/4(K), Working MOSFET3/4(K), Working MOSFET1/4(K)
  Product5/1 -> Working MOSFET3/2(Vgs)
  0.5+0.333 phase/1 -> Switch 5/2
  Gate Driver/3(Switch 3 PWM) -> Product5/2
  Gate Driver/6(Switch 6 PWM) -> Product6/2
  Working MOSFET5/1(Vout) -> AB/2, Vab/2, -Vb/1  "-Vb"
  Gate Driver/5(Switch 5 PWM) -> Product2/2
  Working MOSFET1/1(Vout) -> AB/1, Vab/1, Va/1  "Va"
  0 phase/1 -> Switch 1/2
  Gate Driver/2(Switch 2 PWM) -> Product4/2
  Gate Driver/4(Switch 4 PWM) -> Product1/2
  BC/1 -> Delta Motor/2(Vbc), Voltages/2, Voltage BC/1  "Voltage BC"
  CA/1 -> Delta Motor/3(Vca), Voltages/3, Voltage CA/1  "Voltage CA"
  Working MOSFET3/1(Vout) -> CA/1, Vca/1, Vc/1  "Vc"
  Gate Driver/1(Switch 1 PWM) -> Product3/2
  Vth/1 -> Working MOSFET4/5(Vth), Working MOSFET5/5(Vth), Working MOSFET2/5(Vth), Working MOSFET6/5(Vth), Working MOSFET3/5(Vth), Working MOSFET1/5(Vth)
  Product1/1 -> Working MOSFET4/2(Vgs)
  0.333 phase/1 -> Switch 2/2
  Sum1/1 -> Voltage AB (SW1 to SW5)/1
  0.5 phase/1 -> Switch 4/2
  Switch 1/1 -> Sum1/1
  Working MOSFET2/1(Vout) -> BC/1, Vbc/1, Vb/1  "Vb"
  Switch 6/1 -> Out4/1
  Switch 2/1 -> Out1/1
  Switch 4/1 -> Out3/1
  Product2/1 -> Working MOSFET5/2(Vgs)
  Switch 3/1 -> Out2/1
  +Vs/1 -> Switch 6/1, Switch 3/1, Switch 5/1, Switch 2/1, Switch 4/1, Switch 1/1
  0.666 phase/1 -> Switch 3/2
  0.5+0.666 phase/1 -> Switch 6/2
  -Vs/1 -> Switch 1/3, Switch 6/3, Switch 3/3, Switch 2/3, Switch 5/3, Switch 4/3
  Rds ON/1 -> Working MOSFET1/3(R), Working MOSFET4/3(R), Working MOSFET3/3(R), Working MOSFET6/3(R), Working MOSFET5/3(R), Working MOSFET2/3(R)
  Product4/1 -> Working MOSFET2/2(Vgs)
  Product3/1 -> Working MOSFET1/2(Vgs)
  Product6/1 -> Working MOSFET6/2(Vgs)
  Delta Motor/1(M2_Current) -> M2Current/1

== system Motor_Quadcopter_Combined_Current/Motor_Fault/Subsystem ==
  In1 : Inport
  Add5 : Sum
  Band-Limited White Noise4 : simulink/Sources/Band-Limited White Noise  Cov=[0.0001]  Ts=0.01  seed=[46561]
  Out1 : Outport
  wires:
  Band-Limited White Noise4/1 -> Add5/2
  In1/1 -> Add5/1
  Add5/1 -> Out1/1

== system Motor_Quadcopter_Combined_Current/Motor_Fault/Subsystem1 ==
  In1 : Inport
  Add5 : Sum
  Band-Limited White Noise4 : simulink/Sources/Band-Limited White Noise  Cov=[0.0007]  Ts=0.01  seed=[465]
  Out1 : Outport
  wires:
  Band-Limited White Noise4/1 -> Add5/2
  In1/1 -> Add5/1
  Add5/1 -> Out1/1

== system Motor_Quadcopter_Combined_Current/Motor_Fault/Subsystem2 ==
  In1 : Inport
  Add5 : Sum
  Band-Limited White Noise4 : simulink/Sources/Band-Limited White Noise  Cov=[0.0001]  Ts=0.01  seed=[1765]
  Out1 : Outport
  wires:
  Band-Limited White Noise4/1 -> Add5/2
  In1/1 -> Add5/1
  Add5/1 -> Out1/1

== system Motor_Quadcopter_Combined_Current/Motor_Fault/Subsystem3 ==
  In1 : Inport
  Add5 : Sum
  Band-Limited White Noise4 : simulink/Sources/Band-Limited White Noise  Cov=[0.0004]  Ts=0.01  seed=[3435]
  Out1 : Outport
  wires:
  Band-Limited White Noise4/1 -> Add5/2
  In1/1 -> Add5/1
  Add5/1 -> Out1/1

== system Motor_Quadcopter_Combined_Current/Motor_Fault/Subsystem4 ==
  In1 : Inport
  Add5 : Sum
  Band-Limited White Noise4 : simulink/Sources/Band-Limited White Noise  Cov=[0.0002]  Ts=0.01  seed=[43]
  Out1 : Outport
  wires:
  Band-Limited White Noise4/1 -> Add5/2
  In1/1 -> Add5/1
  Add5/1 -> Out1/1

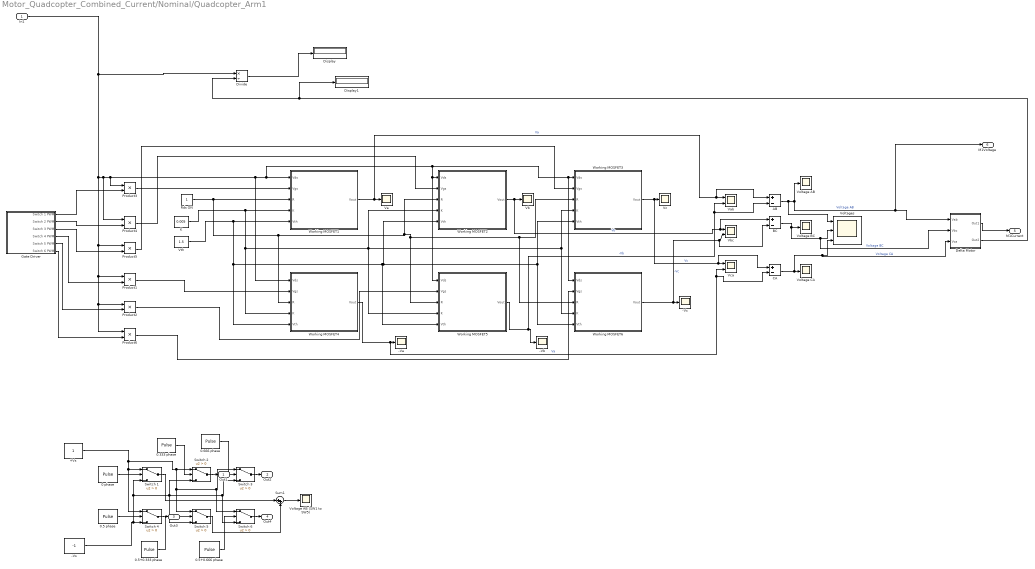
== system Motor_Quadcopter_Combined_Current/Nominal/Quadcopter_Arm1 ==
  In1 : Inport
  +Vs : Constant
  -Va : Scope
  -Vb : Scope
  -Vc : Scope
  -Vs : Constant  Value=-1
  0 phase : DiscretePulseGenerator  PulseType=Time based  Period=1  PulseWidth=50
  0.333 phase : DiscretePulseGenerator  PulseType=Time based  Period=1  PulseWidth=50  PhaseDelay=1/3
  0.5 phase : DiscretePulseGenerator  PulseType=Time based  Period=1  PulseWidth=50  PhaseDelay=.5
  0.5+0.333 phase : DiscretePulseGenerator  PulseType=Time based  Period=1  PulseWidth=50  PhaseDelay=0.5 + 1/3
  0.5+0.666 phase : DiscretePulseGenerator  PulseType=Time based  Period=1  PulseWidth=50  PhaseDelay=2/3+0.5
  0.666 phase : DiscretePulseGenerator  PulseType=Time based  Period=1  PulseWidth=50  PhaseDelay=2/3
  AB : Sum  Inputs=+-
  BC : Sum  Inputs=+-
  CA : Sum  Inputs=+-
  Delta Motor : Subsystem
  Display : Display
  Display1 : Display
  Divide : Product  Inputs=*/
  Gate Driver : Subsystem
  K : Constant  Value=0.005
  Product{1..6} (6 alike) : Product
  Rds ON : Constant
  Sum1 : Sum  Inputs=|++
  Switch {1..6} (6 alike) : Switch  Criteria=u2 > Threshold
  Va : Scope
  Vab : Scope  NumInputPorts=2
  Vb : Scope
  Vbc : Scope  NumInputPorts=2
  Vc : Scope
  Vca : Scope  NumInputPorts=2
  Voltage AB : Scope
  Voltage AB (SW1 to SW5) : Scope
  Voltage BC : Scope
  Voltage CA : Scope
  Voltages : Scope  NumInputPorts=3
  Vth : Constant  Value=1.5
  Working MOSFET1 : MATLAB Function  TreatAsAtomicUnit=on
  Working MOSFET2 : MATLAB Function  TreatAsAtomicUnit=on
  Working MOSFET3 : MATLAB Function  TreatAsAtomicUnit=on
  Working MOSFET4 : MATLAB Function  TreatAsAtomicUnit=on
  Working MOSFET5 : MATLAB Function  TreatAsAtomicUnit=on
  Working MOSFET6 : MATLAB Function  TreatAsAtomicUnit=on
  Out1 : Outport
  Out2 : Outport  Port=2
  Out3 : Outport  Port=3
  Out4 : Outport  Port=4
  M1Current : Outport  Port=5
  M1Voltage : Outport  Port=6
  wires:
  Switch 5/1 -> Sum1/2
  Working MOSFET4/1(Vout) -> CA/2, Vca/2, -Va/1  "Va"
  Working MOSFET6/1(Vout) -> BC/2, Vbc/2, -Vc/1  "-Vc"
  AB/1 -> Voltages/1, M1Voltage/1, Delta Motor/1(Vab), Voltage AB/1  "Voltage AB"
  In1/1 -> Divide/1, Product6/1, Product2/1, Product1/1, Product5/1, Product4/1, Working MOSFET4/1(Vds), Working MOSFET6/1(Vds), Working MOSFET3/1(Vds), Working MOSFET5/1(Vds), Working MOSFET2/1(Vds), Working MOSFET1/1(Vds), Product3/1
  K/1 -> Working MOSFET4/4(K), Working MOSFET5/4(K), Working MOSFET2/4(K), Working MOSFET6/4(K), Working MOSFET3/4(K), Working MOSFET1/4(K)
  Product5/1 -> Working MOSFET3/2(Vgs)
  0.5+0.333 phase/1 -> Switch 5/2
  Gate Driver/3(Switch 3 PWM) -> Product5/2
  Gate Driver/6(Switch 6 PWM) -> Product6/2
  Working MOSFET5/1(Vout) -> AB/2, Vab/2, -Vb/1  "-Vb"
  Gate Driver/5(Switch 5 PWM) -> Product2/2
  Working MOSFET1/1(Vout) -> AB/1, Vab/1, Va/1  "Va"
  0 phase/1 -> Switch 1/2
  Gate Driver/2(Switch 2 PWM) -> Product4/2
  Gate Driver/4(Switch 4 PWM) -> Product1/2
  BC/1 -> Delta Motor/2(Vbc), Voltages/2, Voltage BC/1  "Voltage BC"
  CA/1 -> Delta Motor/3(Vca), Voltages/3, Voltage CA/1  "Voltage CA"
  Working MOSFET3/1(Vout) -> CA/1, Vca/1, Vc/1  "Vc"
  Gate Driver/1(Switch 1 PWM) -> Product3/2
  Vth/1 -> Working MOSFET4/5(Vth), Working MOSFET5/5(Vth), Working MOSFET2/5(Vth), Working MOSFET6/5(Vth), Working MOSFET3/5(Vth), Working MOSFET1/5(Vth)
  Product1/1 -> Working MOSFET4/2(Vgs)
  0.333 phase/1 -> Switch 2/2
  Sum1/1 -> Voltage AB (SW1 to SW5)/1
  0.5 phase/1 -> Switch 4/2
  Switch 1/1 -> Sum1/1
  Working MOSFET2/1(Vout) -> BC/1, Vbc/1, Vb/1  "Vb"
  Switch 6/1 -> Out4/1
  Switch 2/1 -> Out1/1
  Switch 4/1 -> Out3/1
  Product2/1 -> Working MOSFET5/2(Vgs)
  Switch 3/1 -> Out2/1
  +Vs/1 -> Switch 6/1, Switch 3/1, Switch 5/1, Switch 2/1, Switch 4/1, Switch 1/1
  0.666 phase/1 -> Switch 3/2
  0.5+0.666 phase/1 -> Switch 6/2
  -Vs/1 -> Switch 1/3, Switch 6/3, Switch 3/3, Switch 2/3, Switch 5/3, Switch 4/3
  Rds ON/1 -> Working MOSFET1/3(R), Working MOSFET4/3(R), Working MOSFET3/3(R), Working MOSFET6/3(R), Working MOSFET5/3(R), Working MOSFET2/3(R)
  Product4/1 -> Working MOSFET2/2(Vgs)
  Product3/1 -> Working MOSFET1/2(Vgs)
  Product6/1 -> Working MOSFET6/2(Vgs)
  Delta Motor/1(Out1) -> M1Current/1
  Divide/1 -> Display/1
  Delta Motor/2(Out2) -> Display1/1, Divide/2

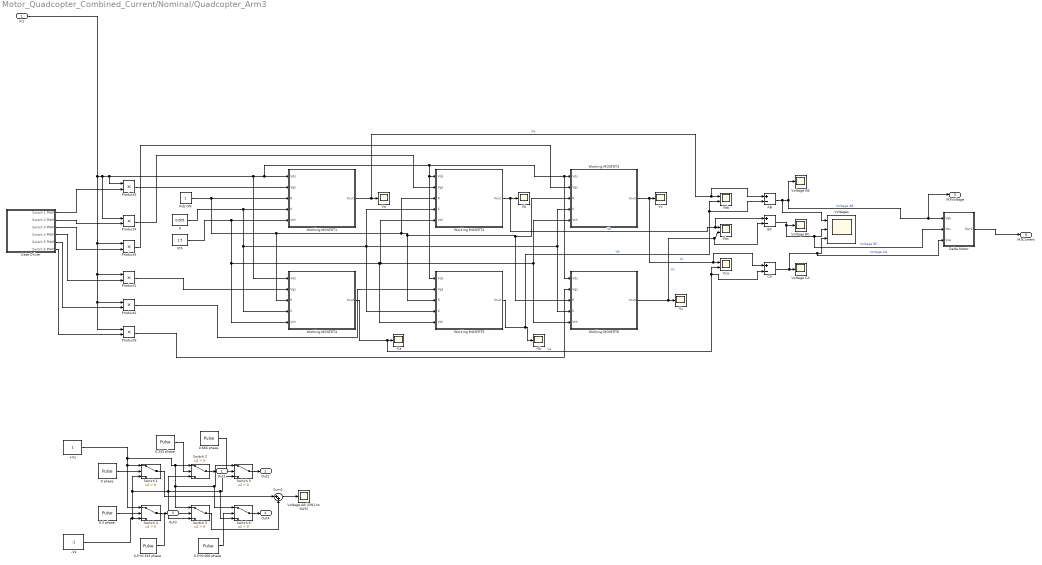
== system Motor_Quadcopter_Combined_Current/Nominal/Quadcopter_Arm3 ==
  In1 : Inport
  +Vs : Constant
  -Va : Scope
  -Vb : Scope
  -Vc : Scope
  -Vs : Constant  Value=-1
  0 phase : DiscretePulseGenerator  PulseType=Time based  Period=1  PulseWidth=50
  0.333 phase : DiscretePulseGenerator  PulseType=Time based  Period=1  PulseWidth=50  PhaseDelay=1/3
  0.5 phase : DiscretePulseGenerator  PulseType=Time based  Period=1  PulseWidth=50  PhaseDelay=.5
  0.5+0.333 phase : DiscretePulseGenerator  PulseType=Time based  Period=1  PulseWidth=50  PhaseDelay=0.5 + 1/3
  0.5+0.666 phase : DiscretePulseGenerator  PulseType=Time based  Period=1  PulseWidth=50  PhaseDelay=2/3+0.5
  0.666 phase : DiscretePulseGenerator  PulseType=Time based  Period=1  PulseWidth=50  PhaseDelay=2/3
  AB : Sum  Inputs=+-
  BC : Sum  Inputs=+-
  CA : Sum  Inputs=+-
  Delta Motor : Subsystem
  Gate Driver : Subsystem
  K : Constant  Value=0.005
  Product{1..6} (6 alike) : Product
  Rds ON : Constant
  Sum1 : Sum  Inputs=|++
  Switch {1..6} (6 alike) : Switch  Criteria=u2 > Threshold
  Va : Scope
  Vab : Scope  NumInputPorts=2
  Vb : Scope
  Vbc : Scope  NumInputPorts=2
  Vc : Scope
  Vca : Scope  NumInputPorts=2
  Voltage AB : Scope
  Voltage AB (SW1 to SW5) : Scope
  Voltage BC : Scope
  Voltage CA : Scope
  Voltages : Scope  NumInputPorts=3
  Vth : Constant  Value=1.5
  Working MOSFET1 : MATLAB Function  TreatAsAtomicUnit=on
  Working MOSFET2 : MATLAB Function  TreatAsAtomicUnit=on
  Working MOSFET3 : MATLAB Function  TreatAsAtomicUnit=on
  Working MOSFET4 : MATLAB Function  TreatAsAtomicUnit=on
  Working MOSFET5 : MATLAB Function  TreatAsAtomicUnit=on
  Working MOSFET6 : MATLAB Function  TreatAsAtomicUnit=on
  Out1 : Outport
  Out2 : Outport  Port=2
  Out3 : Outport  Port=3
  Out4 : Outport  Port=4
  M3Voltage : Outport  Port=5
  M3Current : Outport  Port=6
  wires:
  Switch 5/1 -> Sum1/2
  Working MOSFET4/1(Vout) -> CA/2, Vca/2, -Va/1  "Va"
  Working MOSFET6/1(Vout) -> BC/2, Vbc/2, -Vc/1  "-Vc"
  AB/1 -> Voltages/1, M3Voltage/1, Delta Motor/1(Vab), Voltage AB/1  "Voltage AB"
  In1/1 -> Product6/1, Product2/1, Product1/1, Product5/1, Product4/1, Working MOSFET4/1(Vds), Working MOSFET6/1(Vds), Working MOSFET3/1(Vds), Working MOSFET5/1(Vds), Working MOSFET2/1(Vds), Working MOSFET1/1(Vds), Product3/1
  K/1 -> Working MOSFET4/4(K), Working MOSFET5/4(K), Working MOSFET2/4(K), Working MOSFET6/4(K), Working MOSFET3/4(K), Working MOSFET1/4(K)
  Product5/1 -> Working MOSFET3/2(Vgs)
  0.5+0.333 phase/1 -> Switch 5/2
  Gate Driver/3(Switch 3 PWM) -> Product5/2
  Gate Driver/6(Switch 6 PWM) -> Product6/2
  Working MOSFET5/1(Vout) -> AB/2, Vab/2, -Vb/1  "-Vb"
  Gate Driver/5(Switch 5 PWM) -> Product2/2
  Working MOSFET1/1(Vout) -> AB/1, Vab/1, Va/1  "Va"
  0 phase/1 -> Switch 1/2
  Gate Driver/2(Switch 2 PWM) -> Product4/2
  Gate Driver/4(Switch 4 PWM) -> Product1/2
  BC/1 -> Delta Motor/2(Vbc), Voltages/2, Voltage BC/1  "Voltage BC"
  CA/1 -> Delta Motor/3(Vca), Voltages/3, Voltage CA/1  "Voltage CA"
  Working MOSFET3/1(Vout) -> CA/1, Vca/1, Vc/1  "Vc"
  Gate Driver/1(Switch 1 PWM) -> Product3/2
  Vth/1 -> Working MOSFET4/5(Vth), Working MOSFET5/5(Vth), Working MOSFET2/5(Vth), Working MOSFET6/5(Vth), Working MOSFET3/5(Vth), Working MOSFET1/5(Vth)
  Product1/1 -> Working MOSFET4/2(Vgs)
  0.333 phase/1 -> Switch 2/2
  Sum1/1 -> Voltage AB (SW1 to SW5)/1
  0.5 phase/1 -> Switch 4/2
  Switch 1/1 -> Sum1/1
  Working MOSFET2/1(Vout) -> BC/1, Vbc/1, Vb/1  "Vb"
  Switch 6/1 -> Out4/1
  Switch 2/1 -> Out1/1
  Switch 4/1 -> Out3/1
  Product2/1 -> Working MOSFET5/2(Vgs)
  Switch 3/1 -> Out2/1
  +Vs/1 -> Switch 6/1, Switch 3/1, Switch 5/1, Switch 2/1, Switch 4/1, Switch 1/1
  0.666 phase/1 -> Switch 3/2
  0.5+0.666 phase/1 -> Switch 6/2
  -Vs/1 -> Switch 1/3, Switch 6/3, Switch 3/3, Switch 2/3, Switch 5/3, Switch 4/3
  Rds ON/1 -> Working MOSFET1/3(R), Working MOSFET4/3(R), Working MOSFET3/3(R), Working MOSFET6/3(R), Working MOSFET5/3(R), Working MOSFET2/3(R)
  Product4/1 -> Working MOSFET2/2(Vgs)
  Product3/1 -> Working MOSFET1/2(Vgs)
  Product6/1 -> Working MOSFET6/2(Vgs)
  Delta Motor/1(Out1) -> M3Current/1

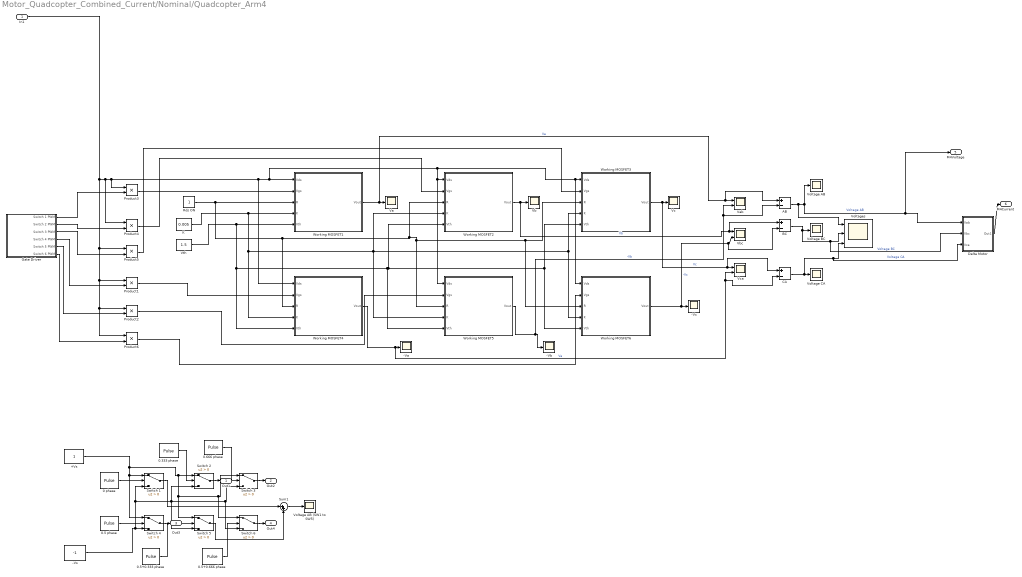
== system Motor_Quadcopter_Combined_Current/Nominal/Quadcopter_Arm4 ==
  In1 : Inport
  +Vs : Constant
  -Va : Scope
  -Vb : Scope
  -Vc : Scope
  -Vs : Constant  Value=-1
  0 phase : DiscretePulseGenerator  PulseType=Time based  Period=1  PulseWidth=50
  0.333 phase : DiscretePulseGenerator  PulseType=Time based  Period=1  PulseWidth=50  PhaseDelay=1/3
  0.5 phase : DiscretePulseGenerator  PulseType=Time based  Period=1  PulseWidth=50  PhaseDelay=.5
  0.5+0.333 phase : DiscretePulseGenerator  PulseType=Time based  Period=1  PulseWidth=50  PhaseDelay=0.5 + 1/3
  0.5+0.666 phase : DiscretePulseGenerator  PulseType=Time based  Period=1  PulseWidth=50  PhaseDelay=2/3+0.5
  0.666 phase : DiscretePulseGenerator  PulseType=Time based  Period=1  PulseWidth=50  PhaseDelay=2/3
  AB : Sum  Inputs=+-
  BC : Sum  Inputs=+-
  CA : Sum  Inputs=+-
  Delta Motor : Subsystem
  Gate Driver : Subsystem
  K : Constant  Value=0.005
  Product{1..6} (6 alike) : Product
  Rds ON : Constant
  Sum1 : Sum  Inputs=|++
  Switch {1..6} (6 alike) : Switch  Criteria=u2 > Threshold
  Va : Scope
  Vab : Scope  NumInputPorts=2
  Vb : Scope
  Vbc : Scope  NumInputPorts=2
  Vc : Scope
  Vca : Scope  NumInputPorts=2
  Voltage AB : Scope
  Voltage AB (SW1 to SW5) : Scope
  Voltage BC : Scope
  Voltage CA : Scope
  Voltages : Scope  NumInputPorts=3
  Vth : Constant  Value=1.5
  Working MOSFET1 : MATLAB Function  TreatAsAtomicUnit=on
  Working MOSFET2 : MATLAB Function  TreatAsAtomicUnit=on
  Working MOSFET3 : MATLAB Function  TreatAsAtomicUnit=on
  Working MOSFET4 : MATLAB Function  TreatAsAtomicUnit=on
  Working MOSFET5 : MATLAB Function  TreatAsAtomicUnit=on
  Working MOSFET6 : MATLAB Function  TreatAsAtomicUnit=on
  Out1 : Outport
  Out2 : Outport  Port=2
  Out3 : Outport  Port=3
  Out4 : Outport  Port=4
  M4Voltage : Outport  Port=5
  M4Current : Outport  Port=6
  wires:
  Switch 5/1 -> Sum1/2
  Working MOSFET4/1(Vout) -> CA/2, Vca/2, -Va/1  "Va"
  Working MOSFET6/1(Vout) -> BC/2, Vbc/2, -Vc/1  "-Vc"
  AB/1 -> Voltages/1, M4Voltage/1, Delta Motor/1(Vab), Voltage AB/1  "Voltage AB"
  In1/1 -> Product6/1, Product2/1, Product1/1, Product5/1, Product4/1, Working MOSFET4/1(Vds), Working MOSFET6/1(Vds), Working MOSFET3/1(Vds), Working MOSFET5/1(Vds), Working MOSFET2/1(Vds), Working MOSFET1/1(Vds), Product3/1
  K/1 -> Working MOSFET4/4(K), Working MOSFET5/4(K), Working MOSFET2/4(K), Working MOSFET6/4(K), Working MOSFET3/4(K), Working MOSFET1/4(K)
  Product5/1 -> Working MOSFET3/2(Vgs)
  0.5+0.333 phase/1 -> Switch 5/2
  Gate Driver/3(Switch 3 PWM) -> Product5/2
  Gate Driver/6(Switch 6 PWM) -> Product6/2
  Working MOSFET5/1(Vout) -> AB/2, Vab/2, -Vb/1  "-Vb"
  Gate Driver/5(Switch 5 PWM) -> Product2/2
  Working MOSFET1/1(Vout) -> AB/1, Vab/1, Va/1  "Va"
  0 phase/1 -> Switch 1/2
  Gate Driver/2(Switch 2 PWM) -> Product4/2
  Gate Driver/4(Switch 4 PWM) -> Product1/2
  BC/1 -> Delta Motor/2(Vbc), Voltages/2, Voltage BC/1  "Voltage BC"
  CA/1 -> Delta Motor/3(Vca), Voltages/3, Voltage CA/1  "Voltage CA"
  Working MOSFET3/1(Vout) -> CA/1, Vca/1, Vc/1  "Vc"
  Gate Driver/1(Switch 1 PWM) -> Product3/2
  Vth/1 -> Working MOSFET4/5(Vth), Working MOSFET5/5(Vth), Working MOSFET2/5(Vth), Working MOSFET6/5(Vth), Working MOSFET3/5(Vth), Working MOSFET1/5(Vth)
  Product1/1 -> Working MOSFET4/2(Vgs)
  0.333 phase/1 -> Switch 2/2
  Sum1/1 -> Voltage AB (SW1 to SW5)/1
  0.5 phase/1 -> Switch 4/2
  Switch 1/1 -> Sum1/1
  Working MOSFET2/1(Vout) -> BC/1, Vbc/1, Vb/1  "Vb"
  Switch 6/1 -> Out4/1
  Switch 2/1 -> Out1/1
  Switch 4/1 -> Out3/1
  Product2/1 -> Working MOSFET5/2(Vgs)
  Switch 3/1 -> Out2/1
  +Vs/1 -> Switch 6/1, Switch 3/1, Switch 5/1, Switch 2/1, Switch 4/1, Switch 1/1
  0.666 phase/1 -> Switch 3/2
  0.5+0.666 phase/1 -> Switch 6/2
  -Vs/1 -> Switch 1/3, Switch 6/3, Switch 3/3, Switch 2/3, Switch 5/3, Switch 4/3
  Rds ON/1 -> Working MOSFET1/3(R), Working MOSFET4/3(R), Working MOSFET3/3(R), Working MOSFET6/3(R), Working MOSFET5/3(R), Working MOSFET2/3(R)
  Product4/1 -> Working MOSFET2/2(Vgs)
  Product3/1 -> Working MOSFET1/2(Vgs)
  Product6/1 -> Working MOSFET6/2(Vgs)
  Delta Motor/1(Out1) -> M4Current/1

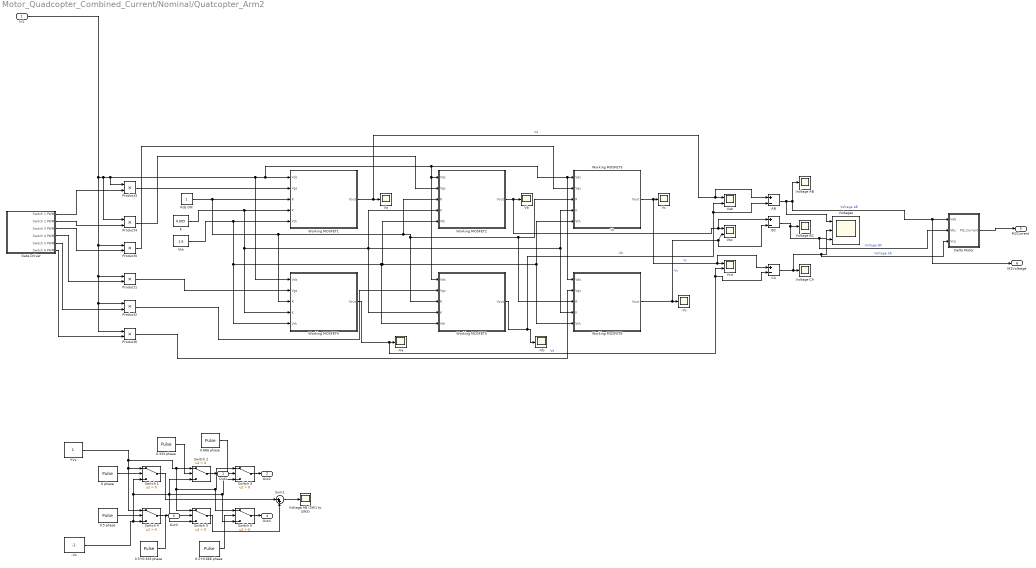
== system Motor_Quadcopter_Combined_Current/Nominal/Quatcopter_Arm2 ==
  In1 : Inport
  +Vs : Constant
  -Va : Scope
  -Vb : Scope
  -Vc : Scope
  -Vs : Constant  Value=-1
  0 phase : DiscretePulseGenerator  PulseType=Time based  Period=1  PulseWidth=50
  0.333 phase : DiscretePulseGenerator  PulseType=Time based  Period=1  PulseWidth=50  PhaseDelay=1/3
  0.5 phase : DiscretePulseGenerator  PulseType=Time based  Period=1  PulseWidth=50  PhaseDelay=.5
  0.5+0.333 phase : DiscretePulseGenerator  PulseType=Time based  Period=1  PulseWidth=50  PhaseDelay=0.5 + 1/3
  0.5+0.666 phase : DiscretePulseGenerator  PulseType=Time based  Period=1  PulseWidth=50  PhaseDelay=2/3+0.5
  0.666 phase : DiscretePulseGenerator  PulseType=Time based  Period=1  PulseWidth=50  PhaseDelay=2/3
  AB : Sum  Inputs=+-
  BC : Sum  Inputs=+-
  CA : Sum  Inputs=+-
  Delta Motor : Subsystem
  Gate Driver : Subsystem
  K : Constant  Value=0.005
  Product{1..6} (6 alike) : Product
  Rds ON : Constant
  Sum1 : Sum  Inputs=|++
  Switch {1..6} (6 alike) : Switch  Criteria=u2 > Threshold
  Va : Scope
  Vab : Scope  NumInputPorts=2
  Vb : Scope
  Vbc : Scope  NumInputPorts=2
  Vc : Scope
  Vca : Scope  NumInputPorts=2
  Voltage AB : Scope
  Voltage AB (SW1 to SW5) : Scope
  Voltage BC : Scope
  Voltage CA : Scope
  Voltages : Scope  NumInputPorts=3
  Vth : Constant  Value=1.5
  Working MOSFET1 : MATLAB Function  TreatAsAtomicUnit=on
  Working MOSFET2 : MATLAB Function  TreatAsAtomicUnit=on
  Working MOSFET3 : MATLAB Function  TreatAsAtomicUnit=on
  Working MOSFET4 : MATLAB Function  TreatAsAtomicUnit=on
  Working MOSFET5 : MATLAB Function  TreatAsAtomicUnit=on
  Working MOSFET6 : MATLAB Function  TreatAsAtomicUnit=on
  Out1 : Outport
  Out2 : Outport  Port=2
  Out3 : Outport  Port=3
  Out4 : Outport  Port=4
  M2Current : Outport  Port=5
  M2Voltatge : Outport  Port=6
  wires:
  Switch 5/1 -> Sum1/2
  Working MOSFET4/1(Vout) -> CA/2, Vca/2, -Va/1  "Va"
  Working MOSFET6/1(Vout) -> BC/2, Vbc/2, -Vc/1  "-Vc"
  AB/1 -> Voltages/1, M2Voltatge/1, Delta Motor/1(Vab), Voltage AB/1  "Voltage AB"
  In1/1 -> Product6/1, Product2/1, Product1/1, Product5/1, Product4/1, Working MOSFET4/1(Vds), Working MOSFET6/1(Vds), Working MOSFET3/1(Vds), Working MOSFET5/1(Vds), Working MOSFET2/1(Vds), Working MOSFET1/1(Vds), Product3/1
  K/1 -> Working MOSFET4/4(K), Working MOSFET5/4(K), Working MOSFET2/4(K), Working MOSFET6/4(K), Working MOSFET3/4(K), Working MOSFET1/4(K)
  Product5/1 -> Working MOSFET3/2(Vgs)
  0.5+0.333 phase/1 -> Switch 5/2
  Gate Driver/3(Switch 3 PWM) -> Product5/2
  Gate Driver/6(Switch 6 PWM) -> Product6/2
  Working MOSFET5/1(Vout) -> AB/2, Vab/2, -Vb/1  "-Vb"
  Gate Driver/5(Switch 5 PWM) -> Product2/2
  Working MOSFET1/1(Vout) -> AB/1, Vab/1, Va/1  "Va"
  0 phase/1 -> Switch 1/2
  Gate Driver/2(Switch 2 PWM) -> Product4/2
  Gate Driver/4(Switch 4 PWM) -> Product1/2
  BC/1 -> Delta Motor/2(Vbc), Voltages/2, Voltage BC/1  "Voltage BC"
  CA/1 -> Delta Motor/3(Vca), Voltages/3, Voltage CA/1  "Voltage CA"
  Working MOSFET3/1(Vout) -> CA/1, Vca/1, Vc/1  "Vc"
  Gate Driver/1(Switch 1 PWM) -> Product3/2
  Vth/1 -> Working MOSFET4/5(Vth), Working MOSFET5/5(Vth), Working MOSFET2/5(Vth), Working MOSFET6/5(Vth), Working MOSFET3/5(Vth), Working MOSFET1/5(Vth)
  Product1/1 -> Working MOSFET4/2(Vgs)
  0.333 phase/1 -> Switch 2/2
  Sum1/1 -> Voltage AB (SW1 to SW5)/1
  0.5 phase/1 -> Switch 4/2
  Switch 1/1 -> Sum1/1
  Working MOSFET2/1(Vout) -> BC/1, Vbc/1, Vb/1  "Vb"
  Switch 6/1 -> Out4/1
  Switch 2/1 -> Out1/1
  Switch 4/1 -> Out3/1
  Product2/1 -> Working MOSFET5/2(Vgs)
  Switch 3/1 -> Out2/1
  +Vs/1 -> Switch 6/1, Switch 3/1, Switch 5/1, Switch 2/1, Switch 4/1, Switch 1/1
  0.666 phase/1 -> Switch 3/2
  0.5+0.666 phase/1 -> Switch 6/2
  -Vs/1 -> Switch 1/3, Switch 6/3, Switch 3/3, Switch 2/3, Switch 5/3, Switch 4/3
  Rds ON/1 -> Working MOSFET1/3(R), Working MOSFET4/3(R), Working MOSFET3/3(R), Working MOSFET6/3(R), Working MOSFET5/3(R), Working MOSFET2/3(R)
  Product4/1 -> Working MOSFET2/2(Vgs)
  Product3/1 -> Working MOSFET1/2(Vgs)
  Product6/1 -> Working MOSFET6/2(Vgs)
  Delta Motor/1(M2_Current) -> M2Current/1
